simulink model "model"  (R2015b)
settings: Solver=VariableStepAuto  StartTime=0.0  StopTime=10.0  RelTol=1e-3
libraries: dsparch4 x1, dspsrcs4 x1
settings Model: Creator=Asus  LastModifiedBy=Alex

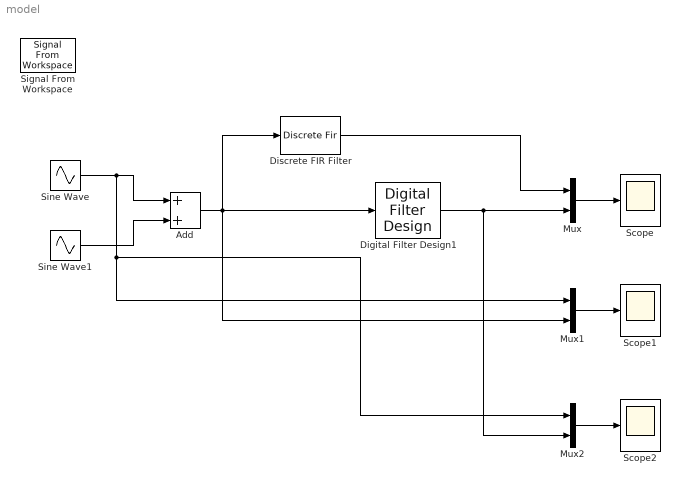
== system model ==
  Add : Sum
  Digital Filter Design1 : dsparch4/Digital Filter Design  mwdsp_browser_bugfix_var=off
  Discrete FIR Filter : DiscreteFir  SampleTime=0.001
  Mux : Mux  Inputs=2
  Mux1 : Mux  Inputs=2
  Mux2 : Mux  Inputs=2
  Scope : Scope
  Scope1 : Scope
  Scope2 : Scope
  Sine Wave : Sin  Amplitude=10  SampleTime=.05  VectorParams1D=off
  Sine Wave1 : Sin  Amplitude=2  Frequency=10  Phase=1  Samples=20  SampleTime=.05  VectorParams1D=off
  Signal From Workspace : dspsrcs4/Signal From Workspace  IOType=siggen  X=1:10  Ts=1  nsamps=1  OutputAfterFinalValue=Setting to zero  ignoreOrWarnInputAndFrameLengths=off  OutputFrames=on
  wires:
  Sine Wave/1 -> Mux2/1, Mux1/1, Add/1
  Sine Wave1/1 -> Add/2
  Mux/1 -> Scope/1
  Discrete FIR Filter/1 -> Mux/1
  Mux1/1 -> Scope1/1
  Mux2/1 -> Scope2/1
  Digital Filter Design1/1 -> Mux2/2, Mux/2
  Add/1 -> Digital Filter Design1/1, Mux1/2, Discrete FIR Filter/1
